simulink model "KSimulator_UR10_3"  (Simulink 9.0)
settings: Solver=FixedStepDiscrete  StartTime=0.0  StopTime=10  FixedStep=0.001  RelTol=1e-3  EnableMultiTasking=on
undefined symbols (not defined in the file or in its folder): SimpleRobotPlotFull
settings Model: SuppressorTable=22 serialization::archive 11 0 6 0 0 0 11 0  Creator=E. Dean  LastModifiedBy=nirnai
settings DataIOCC: LimitDataPoints=on  SignalLoggingSaveFormat=ModelDataLogs
settings OptimizationCC: ExpressionDepthLimit=2147483647
settings DebuggingCC: SolverPrmCheckMsg=warning  FcnCallInpInsideContextMsg=warning  StateNameClashWarn=warning
settings GRTTargetCC: GeneratePreprocessorConditionals=Disable all  CombineOutputUpdateFcns=off  GRTInterface=on
settings ConfigComp: CovSFcnEnable=off

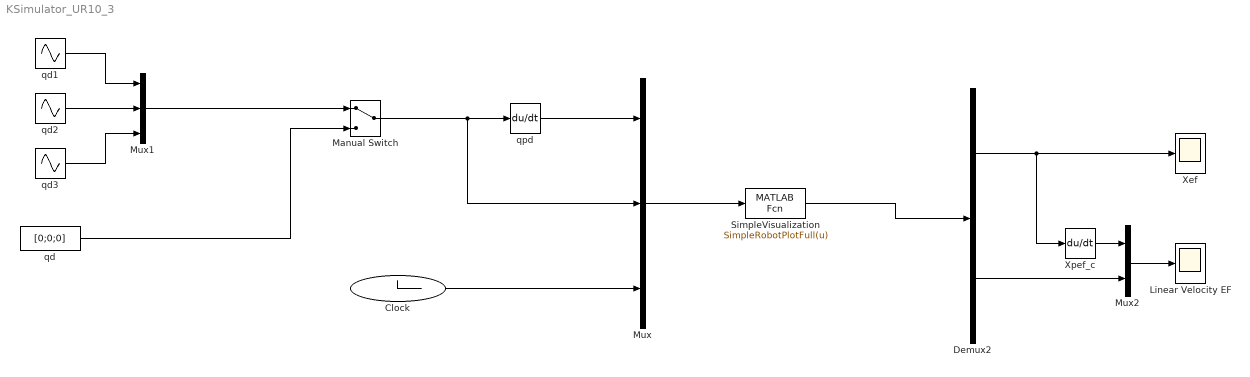
== system KSimulator_UR10_3 ==
  Clock : Clock
  Demux2 : Demux  Outputs=2
  Linear Velocity EF : Scope
  Manual Switch : ManualSwitch
  Mux : Mux  Inputs=3
  Mux1 : Mux  Inputs=3
  Mux2 : Mux  Inputs=2
  SimpleVisualization : MATLABFcn  MATLABFcn=SimpleRobotPlotFull(u)  OutputDimensions=6
  Xef : Scope
  Xpef_c : Derivative
  qd : Constant  Value=[0;0;0]
  qd1 : Sin  SampleTime=0
  qd2 : Sin  SampleTime=0
  qd3 : Sin  SampleTime=0
  qpd : Derivative
  wires:
  Mux/1 -> SimpleVisualization/1
  qd1/1 -> Mux1/1
  qd2/1 -> Mux1/2
  qd3/1 -> Mux1/3
  Mux1/1 -> Manual Switch/1
  qpd/1 -> Mux/1
  SimpleVisualization/1 -> Demux2/1
  Demux2/1 -> Xef/1, Xpef_c/1
  Mux2/1 -> Linear Velocity EF/1
  Xpef_c/1 -> Mux2/1
  Demux2/2 -> Mux2/2
  Clock/1 -> Mux/3
  Manual Switch/1 -> Mux/2, qpd/1
  qd/1 -> Manual Switch/2
